simulink model "FZY1"  (R2018a)
settings: Solver=FixedStepAuto  StartTime=0.0  StopTime=35  FixedStep=0.012  RelTol=1e-3
settings Model: Creator=zhouyu  LastModifiedBy=28213

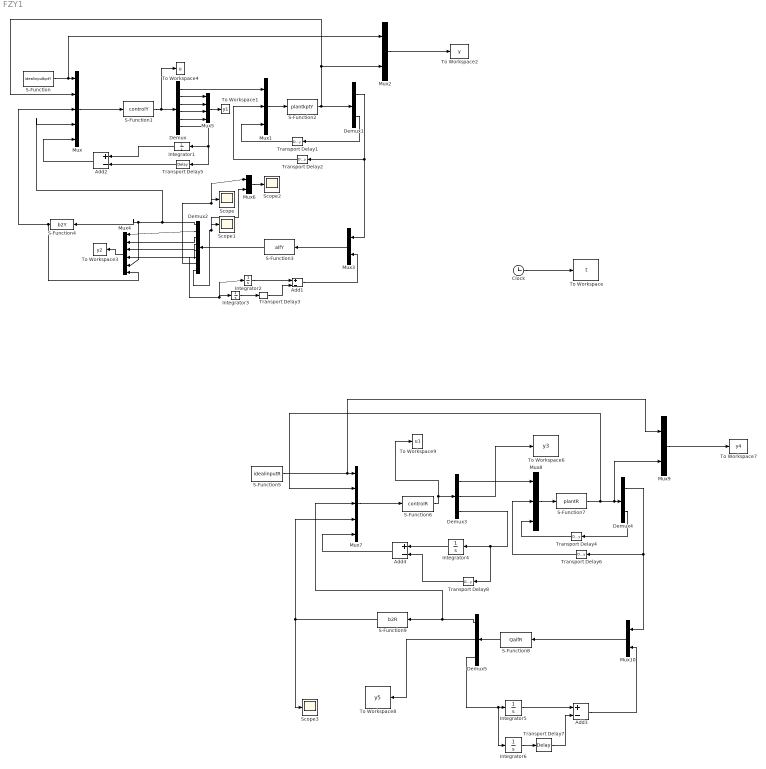
== system FZY1 ==
  Add{1..4} (4 alike) : Sum  Inputs=+-
  Clock : Clock
  Demux : Demux  Outputs=6
  Demux1 : Demux  Outputs=2
  Demux2 : Demux  Outputs=8
  Demux3 : Demux  Outputs=[1 2 1]
  Demux4 : Demux  Outputs=2
  Demux5 : Demux  Outputs=[1 2 1]
  Integrator{1..6} (6 alike) : Integrator
  Mux : Mux  Inputs=5
  Mux1 : Mux  Inputs=3
  Mux{2..3,6,9..10} (5 alike) : Mux  Inputs=2
  Mux4 : Mux  Inputs=6
  Mux5 : Mux
  Mux7 : Mux  Inputs=5
  Mux8 : Mux  Inputs=3
  S-Function : S-Function  FunctionName=idealinputkptY  SFunctionDeploymentMode=off  EnableBusSupport=off
  S-Function1 : S-Function  FunctionName=controlY  SFunctionDeploymentMode=off  EnableBusSupport=off
  S-Function2 : S-Function  FunctionName=plantkptY  SFunctionDeploymentMode=off  EnableBusSupport=off
  S-Function3 : S-Function  FunctionName=alfY  SFunctionDeploymentMode=off  EnableBusSupport=off
  S-Function4 : S-Function  FunctionName=b2Y  SFunctionDeploymentMode=off  EnableBusSupport=off
  S-Function5 : S-Function  FunctionName=idealinputR  SFunctionDeploymentMode=off  EnableBusSupport=off
  S-Function6 : S-Function  FunctionName=controlR  SFunctionDeploymentMode=off  EnableBusSupport=off
  S-Function7 : S-Function  FunctionName=plantR  SFunctionDeploymentMode=off  EnableBusSupport=off
  S-Function8 : S-Function  FunctionName=QalfR  SFunctionDeploymentMode=off  EnableBusSupport=off
  S-Function9 : S-Function  FunctionName=b2R  SFunctionDeploymentMode=off  EnableBusSupport=off
  Scope{,1..3} (4 alike) : Scope
  To Workspace : ToWorkspace  VariableName=t  SampleTime=-1
      settings: Save2DSignal=2-D array (concatenate along first dimension)
  To Workspace1 : ToWorkspace  VariableName=y1  SampleTime=-1
      settings: Save2DSignal=2-D array (concatenate along first dimension)
  To Workspace2 : ToWorkspace  VariableName=y  SampleTime=-1
      settings: Save2DSignal=2-D array (concatenate along first dimension)
  To Workspace3 : ToWorkspace  VariableName=y2  SampleTime=-1
      settings: Save2DSignal=2-D array (concatenate along first dimension)
  To Workspace4 : ToWorkspace  VariableName=u  SampleTime=-1
      settings: Save2DSignal=2-D array (concatenate along first dimension)
  To Workspace6 : ToWorkspace  VariableName=y3  SampleTime=-1
      settings: Save2DSignal=2-D array (concatenate along first dimension)
  To Workspace7 : ToWorkspace  VariableName=y4  SampleTime=-1
      settings: Save2DSignal=2-D array (concatenate along first dimension)
  To Workspace8 : ToWorkspace  VariableName=y5  SampleTime=-1
      settings: Save2DSignal=2-D array (concatenate along first dimension)
  To Workspace9 : ToWorkspace  VariableName=u1  SampleTime=-1
      settings: Save2DSignal=2-D array (concatenate along first dimension)
  Transport Delay1 : TransportDelay  DelayTime=1.5
  Transport Delay2 : TransportDelay
  Transport Delay{3,5,7..8} (4 alike) : TransportDelay  DelayTime=1.6
  Transport Delay4 : TransportDelay  DelayTime=1.5
  Transport Delay6 : TransportDelay
  wires:
  Demux2/3 -> Mux4/2
  Transport Delay2/1 -> Mux1/2
  Integrator1/1 -> Add2/1
  S-Function1/1 -> To Workspace4/1, Demux/1
  Mux2/1 -> To Workspace2/1
  Demux/1 -> Mux1/1
  Transport Delay1/1 -> Mux1/3
  S-Function2/1 -> Mux/2, Mux2/2, Demux1/1
  Demux/2 -> Mux5/1
  Demux/6 -> Transport Delay5/1, Integrator1/1
  Add2/1 -> Mux/5
  Mux1/1 -> S-Function2/1
  Demux2/2 -> Mux4/1
  Clock/1 -> To Workspace/1
  Mux4/1 -> To Workspace3/1
  Demux2/1 -> Mux/4, S-Function4/1, Mux4/5
  Integrator2/1 -> Add1/1
  S-Function/1 -> Mux2/1, Mux/1
  Mux/1 -> S-Function1/1
  Demux1/2 -> Transport Delay1/1
  Transport Delay3/1 -> Add1/2
  Demux1/1 -> Transport Delay2/1, Mux3/1
  Demux2/6 -> Integrator3/1, Integrator2/1
  Integrator3/1 -> Transport Delay3/1
  Add1/1 -> Mux3/2
  Mux5/1 -> To Workspace1/1
  Demux2/4 -> Mux4/3
  Transport Delay5/1 -> Add2/2
  Mux3/1 -> S-Function3/1
  Demux/3 -> Mux5/2
  S-Function3/1 -> Demux2/1
  Demux/4 -> Mux5/3
  Demux/5 -> Mux5/4
  Demux2/5 -> Mux4/4
  S-Function4/1 -> Mux4/6, Mux/3
  Demux2/7 -> Mux6/1, Scope/1
  Demux2/8 -> Mux6/2, Scope1/1
  Mux6/1 -> Scope2/1
  Mux9/1 -> To Workspace7/1
  Integrator4/1 -> Add4/1
  Transport Delay7/1 -> Add3/2
  Mux10/1 -> S-Function8/1
  Demux3/2 -> To Workspace6/1
  S-Function8/1 -> Demux5/1
  Demux4/2 -> Transport Delay4/1
  Add4/1 -> Mux7/5
  S-Function6/1 -> To Workspace9/1, Demux3/1
  Transport Delay4/1 -> Mux8/3
  Demux5/3 -> Integrator6/1, Integrator5/1
  Integrator5/1 -> Add3/1
  Demux5/1 -> Mux7/3, S-Function9/1
  Demux5/2 -> To Workspace8/1
  Integrator6/1 -> Transport Delay7/1
  Demux3/3 -> Transport Delay8/1, Integrator4/1
  S-Function9/1 -> Scope3/1, Mux7/4
  Demux3/1 -> Mux8/1
  Demux4/1 -> Transport Delay6/1, Mux10/1
  Mux8/1 -> S-Function7/1
  Transport Delay8/1 -> Add4/2
  Mux7/1 -> S-Function6/1
  S-Function5/1 -> Mux9/1, Mux7/1
  S-Function7/1 -> Mux9/2, Demux4/1, Mux7/2
  Add3/1 -> Mux10/2
  Transport Delay6/1 -> Mux8/2
